simulink model "plant"  (R2014a)
settings: Solver=ode45  StartTime=0.0  StopTime=simTime  MaxStep=0.001  RelTol=1e-3
settings Model: Creator=Ash  LastModifiedBy=Ash
settings DataIOCC: ExternalInput=Input  LimitDataPoints=off  LoadExternalInput=on  OutputSaveName=r, r_d, s, s_d, r_dd, s_dd

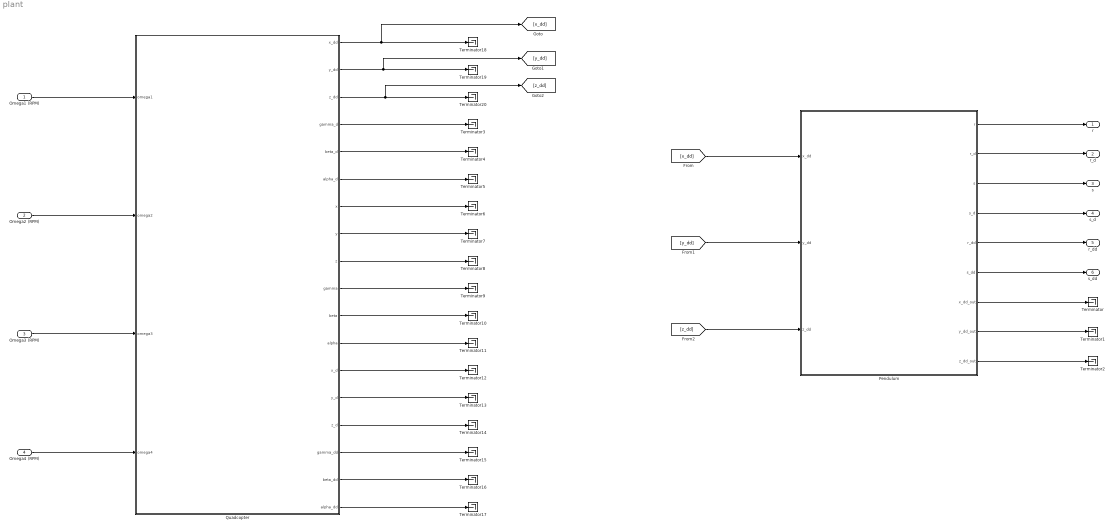
== system plant ==
  Omega1 (RPM) : Inport
  Omega2 (RPM) : Inport  Port=2
  Omega3 (RPM) : Inport  Port=3
  Omega4 (RPM) : Inport  Port=4
  Pendulum : Subsystem
  Quadcopter : Subsystem
  Terminator{,1..20} (21 alike) : Terminator
  r : Outport
  r_d : Outport  Port=2
  s : Outport  Port=3
  s_d : Outport  Port=4
  r_dd : Outport  Port=5
  s_dd : Outport  Port=6
  wires:
  Quadcopter/1(x_dd) -> Terminator18/1, [x_dd]
  Quadcopter/2(y_dd) -> Terminator19/1, [y_dd]
  Omega1 (RPM)/1 -> Quadcopter/1(omega1)
  Omega2 (RPM)/1 -> Quadcopter/2(omega2)
  Omega3 (RPM)/1 -> Quadcopter/3(omega3)
  Omega4 (RPM)/1 -> Quadcopter/4(omega4)
  Quadcopter/3(z_dd) -> Terminator20/1, [z_dd]
  Pendulum/1(r) -> r/1
  Pendulum/2(r_d) -> r_d/1
  Pendulum/4(s_d) -> s_d/1
  Pendulum/3(s) -> s/1
  Pendulum/5(r_dd) -> r_dd/1
  Pendulum/6(s_dd) -> s_dd/1
  [x_dd] -> Pendulum/1(x_dd)
  [y_dd] -> Pendulum/2(y_dd)
  [z_dd] -> Pendulum/3(z_dd)
  Pendulum/7(x_dd_out) -> Terminator/1
  Pendulum/9(z_dd_out) -> Terminator2/1
  Pendulum/8(y_dd_out) -> Terminator1/1
  Quadcopter/4(gamma_d) -> Terminator3/1
  Quadcopter/18(alpha_dd) -> Terminator17/1
  Quadcopter/17(beta_dd) -> Terminator16/1
  Quadcopter/16(gamma_dd) -> Terminator15/1
  Quadcopter/15(z_d) -> Terminator14/1
  Quadcopter/14(y_d) -> Terminator13/1
  Quadcopter/13(x_d) -> Terminator12/1
  Quadcopter/12(alpha) -> Terminator11/1
  Quadcopter/11(beta) -> Terminator10/1
  Quadcopter/10(gamma) -> Terminator9/1
  Quadcopter/9(z) -> Terminator8/1
  Quadcopter/8(y) -> Terminator7/1
  Quadcopter/7(x) -> Terminator6/1
  Quadcopter/6(alpha_d) -> Terminator5/1
  Quadcopter/5(beta_d) -> Terminator4/1

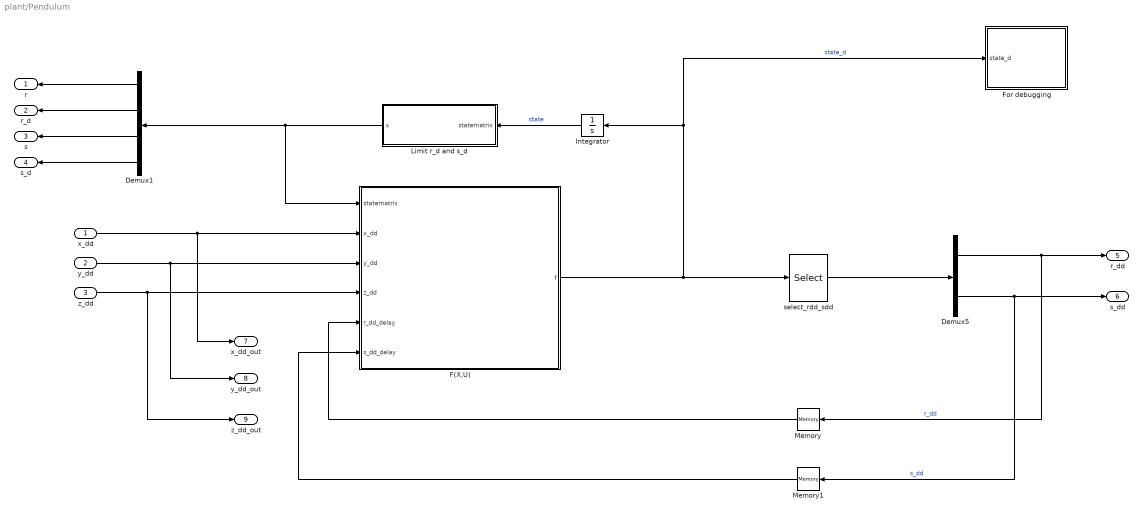
== system plant/Pendulum ==
  x_dd : Inport
  y_dd : Inport  Port=2
  z_dd : Inport  Port=3
  Demux1 : Demux  Outputs=[1 1 1 1]
  Demux5 : Demux  Outputs=[1 1]
  F(X,U) : MATLAB Function  TreatAsAtomicUnit=on
  For debugging : Subsystem
  Integrator : Integrator
  Limit r_d and s_d : MATLAB Function  TreatAsAtomicUnit=on
  Memory : Memory
  Memory1 : Memory
  select_rdd_sdd : Selector  InputPortWidth=4  Indices=[2 4]
  r : Outport
  r_d : Outport  Port=2
  s : Outport  Port=3
  s_d : Outport  Port=4
  r_dd : Outport  Port=5
  s_dd : Outport  Port=6
  x_dd_out : Outport  Port=7
  y_dd_out : Outport  Port=8
  z_dd_out : Outport  Port=9
  wires:
  Memory1/1 -> F(X,U)/6(s_dd_delay)
  Demux5/1 -> r_dd/1, Memory/1  "r_dd"
  Memory/1 -> F(X,U)/5(r_dd_delay)
  select_rdd_sdd/1 -> Demux5/1
  Demux5/2 -> s_dd/1, Memory1/1  "s_dd"
  z_dd/1 -> F(X,U)/4(z_dd), z_dd_out/1
  y_dd/1 -> F(X,U)/3(y_dd), y_dd_out/1
  Demux1/1 -> r/1
  Demux1/2 -> r_d/1
  Demux1/4 -> s_d/1
  Demux1/3 -> s/1
  F(X,U)/1(f) -> For debugging/1(state_d), Integrator/1, select_rdd_sdd/1  "state_d"
  x_dd/1 -> F(X,U)/2(x_dd), x_dd_out/1
  Limit r_d and s_d/1(x) -> F(X,U)/1(statematrix), Demux1/1
  Integrator/1 -> Limit r_d and s_d/1(statematrix)  "state"

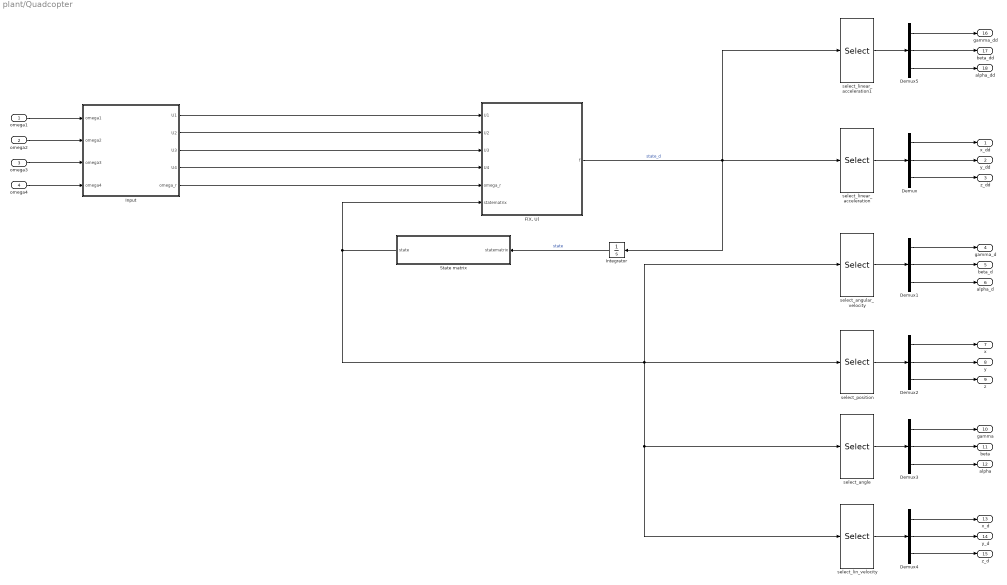
== system plant/Quadcopter ==
  omega1 : Inport
  omega2 : Inport  Port=2
  omega3 : Inport  Port=3
  omega4 : Inport  Port=4
  Demux{,1..5} (6 alike) : Demux  Outputs=[1 1 1]
  "F(X, U)" : MATLAB Function  TreatAsAtomicUnit=on
  Input : MATLAB Function  TreatAsAtomicUnit=on
  Integrator : Integrator
  State matrix : MATLAB Function  TreatAsAtomicUnit=on
  select_angle : Selector  InputPortWidth=12  Indices=[7 9 11]
  select_angular_velocity : Selector  InputPortWidth=12  Indices=[8 10 12]
  select_lin_velocity : Selector  InputPortWidth=12  Indices=[2 4 6]
  select_linear_acceleration : Selector  InputPortWidth=12  Indices=[2 4 6]
  select_linear_acceleration1 : Selector  InputPortWidth=12  Indices=[8 10 12]
  select_position : Selector  InputPortWidth=12  Indices=[1 3 5]
  x_dd : Outport
  y_dd : Outport  Port=2
  z_dd : Outport  Port=3
  gamma_d : Outport  Port=4
  beta_d : Outport  Port=5
  alpha_d : Outport  Port=6
  x : Outport  Port=7
  y : Outport  Port=8
  z : Outport  Port=9
  gamma : Outport  Port=10
  beta : Outport  Port=11
  alpha : Outport  Port=12
  x_d : Outport  Port=13
  y_d : Outport  Port=14
  z_d : Outport  Port=15
  gamma_dd : Outport  Port=16
  beta_dd : Outport  Port=17
  alpha_dd : Outport  Port=18
  wires:
  omega3/1 -> Input/3(omega3)
  omega2/1 -> Input/2(omega2)
  omega1/1 -> Input/1(omega1)
  select_linear_acceleration/1 -> Demux/1
  Demux/1 -> x_dd/1
  Demux/2 -> y_dd/1
  Demux/3 -> z_dd/1
  select_angular_velocity/1 -> Demux1/1
  Demux1/1 -> gamma_d/1
  Demux1/2 -> beta_d/1
  Demux1/3 -> alpha_d/1
  select_position/1 -> Demux2/1
  Demux2/1 -> x/1
  Demux2/2 -> y/1
  Demux2/3 -> z/1
  select_angle/1 -> Demux3/1
  Demux3/1 -> gamma/1
  Demux3/2 -> beta/1
  Demux3/3 -> alpha/1
  Integrator/1 -> State matrix/1(statematrix)  "state"
  select_lin_velocity/1 -> Demux4/1
  Demux4/1 -> x_d/1
  Demux4/2 -> y_d/1
  Demux4/3 -> z_d/1
  omega4/1 -> Input/4(omega4)
  Input/1(U1) -> "F(X, U)"/1(U1)
  Input/2(U2) -> "F(X, U)"/2(U2)
  Input/3(U3) -> "F(X, U)"/3(U3)
  Input/4(U4) -> "F(X, U)"/4(U4)
  Input/5(omega_r) -> "F(X, U)"/5(omega_r)
  "F(X, U)"/1(f) -> select_linear_acceleration1/1, select_linear_acceleration/1, Integrator/1  "state_d"
  select_linear_acceleration1/1 -> Demux5/1
  Demux5/1 -> gamma_dd/1
  Demux5/2 -> beta_dd/1
  Demux5/3 -> alpha_dd/1
  State matrix/1(state) -> "F(X, U)"/6(statematrix), select_angular_velocity/1, select_position/1, select_lin_velocity/1, select_angle/1

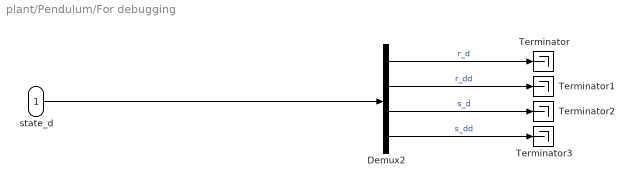
== system plant/Pendulum/For debugging ==
  state_d : Inport
  Demux2 : Demux  Outputs=[1 1 1 1]
  Terminator{,1..3} (4 alike) : Terminator
  wires:
  Demux2/4 -> Terminator3/1  "s_dd"
  Demux2/3 -> Terminator2/1  "s_d"
  Demux2/2 -> Terminator1/1  "r_dd"
  Demux2/1 -> Terminator/1  "r_d"
  state_d/1 -> Demux2/1

== matlab function plant/Quadcopter/State matrix ==
  data: state output; statematrix input
function state = fcn(statematrix)

x = statematrix(1);
x_d = statematrix(2);
y = statematrix(3);
y_d = statematrix(4);
z = statematrix(5);
z_d = statematrix(6);
gamma1 = statematrix(7);
gamma_d = statematrix(8);
beta1 = statematrix(9);
beta_d = statematrix(10);
alpha1 = statematrix(11);
alpha_d = statematrix(12);

gamma = mod(gamma1, 2*3.1416);
beta = mod(beta1, 2*3.1416);
alpha = mod(alpha1, 2*3.1416);

state = [x; x_d; y; y_d; z; z_d; gamma; gamma_d; beta; beta_d; alpha; alpha_d];

== matlab function plant/Quadcopter/F(X, U) ==
  data: U1 input; f output; U2 input; U3 input; U4 input; omega_r input; statematrix input
function f = fcn(U1, U2, U3, U4, omega_r, statematrix)

%syms b d
%syms l_qa l_r m_arm m_body m_rotor h_a h_b h_r r

g = -9.81;
l_qa = 0.25;
l_r = 0.1;
m_arm = 0.01;
m_body = 0.5;
m_rotor = 0.05;
h_a = 0.0025;
h_b = 0.05;
h_r = 0.001;
r = 0.025;

m = m_arm + m_body;
Ixx = (4*m_arm/3) * (h_a^3*(l_qa-r) + h_a*(l_qa^3 - r^3)) + (m_body/3) * (r^3*h_b + r*h_b^3);
Iyy = Ixx;
Izz = (8*m_arm/3) * (l_qa^4 + r^4 - l_qa^3*r - l_qa*r^3) + (2*m_body/3)*r^4;

%Ix = [Ixx 0 0; 0 0 0; 0 0 0];
%Iy = [0 0 0; 0 Iyy 0; 0 0 0];
%Iz = [0 0 0; 0 0 0; 0 0 Izz];
%J = Ix + Iy + Iz;  
Ix = Ixx;
Iy = Iyy;
Iz = Izz;             
J = [Ixx 0 0; 0 Iyy 0; 0 0 Izz];                        % inertia tensor of quadcopter
Jr_x = (m_rotor/3)*(l_r^3*h_r + l_r*h_r^3);
Jr_y = (m_rotor/3)*(l_r^3*h_r + l_r*h_r^3);
Jr_z = (2*m_rotor/3)*l_r^4;
Jr_vector = 4*[Jr_x 0 0; 0 Jr_y 0; 0 0 Jr_z];           % intertia tensor of all 4 rotors
Jr = sqrt(Jr_vector(1,1)^2 + Jr_vector(2,2)^2 + Jr_vector(3,3)^2);

x = statematrix(1);
x_d = statematrix(2);
y = statematrix(3);
y_d = statematrix(4);
z = statematrix(5);
z_d = statematrix(6);
gamma1 = statematrix(7);
gamma_d = statematrix(8);
beta1 = statematrix(9);
beta_d = statematrix(10);
alpha1 = statematrix(11);
alpha_d = statematrix(12);

gamma = mod(gamma1, 2*3.1416);
beta = mod(beta1, 2*3.1416);
alpha = mod(alpha1, 2*3.1416);

L_vector = mtimes(J, [gamma_d; beta_d; alpha_d]);
L = sqrt(L_vector(1)^2 + L_vector(2)^2 + L_vector(3)^2);

f = [x_d; -U1/m*(cos(gamma)*sin(beta)*cos(alpha) + sin(gamma)*sin(alpha)); y_d; -U1/m * (cos(gamma)*sin(alpha)*sin(beta) - sin(gamma)*cos(alpha)); z_d; ((U1/m)*cos(beta)*cos(gamma) + g); gamma_d; (beta_d*alpha_d*((Iy-Iz)/Ix) - (Jr/Ix)*beta_d*omega_r + (L/Ix)*U2); beta_d; (gamma_d*alpha_d*((Iz-Ix)/Iy) + (Jr/Iy)*gamma_d*omega_r + (L/Iy)*U3); alpha_d; (gamma_d*beta_d*((Ix-Iy)/Iz) + (1/Iz)*U4)];

== matlab function plant/Quadcopter/Input ==
  data: omega1 input; omega2 input; omega3 input; U1 output; omega4 input; U2 output; U3 output; U4 output; omega_r output
function [U1, U2, U3, U4, omega_r] = fcn(omega1, omega2 ,omega3, omega4)

%syms b d
b = 3.13e-5;
d = 9e-7;

% convert to rad/s
o1 = omega1 * 2 * pi / 60;
o2 = omega2 * 2 * pi / 60;
o3 = omega3 * 2 * pi / 60;
o4 = omega4 * 2 * pi / 60;

U1 = b*(o1^2 + o2^2 + o3^2 + o4^2);
U2 = b*(-o2^2 + o4^2);
U3 = b*(o1^2 - o3^2);
U4 = d*(o1^2 - o2^2 + o3^2 - o4^2);
omega_r = -o1 + o2 - o3 + o4;

== matlab function plant/Pendulum/F(X,U) ==
  data: statematrix input; x_dd input; y_dd input; z_dd input; r_dd_delay input; s_dd_delay input; f output
function f = fcn(statematrix, x_dd, y_dd, z_dd, r_dd_delay, s_dd_delay)

g = -9.81;
L = 0.4;

r = statematrix(1);
r_d = statematrix(2);
s = statematrix(3);
s_d = statematrix(4);

if ((r^2 + s^2) <= (L^2))
    
    zeta = sqrt(L^2 - r^2 - s^2);
    r_dd = (1/((L^2 - s^2)*zeta)) * ( -r^4*x_dd - (L^2 - s^2)^2*x_dd - 2*r^2*(s*r_d*s_d + (-L^2 + s^2)*x_dd) + r^3*(s_d^2 + s*s_dd_delay - zeta*(g+z_dd)) + r*(-L^2*s*s_dd_delay + s^3*s_dd_delay + s^2*(r_d^2 - zeta*(g+z_dd)) + L^2*(-r_d^2 - s_d^2 + zeta*(g+z_dd))) );
    s_dd = (1/((L^2 - r^2)*zeta)) * ( -s^4*y_dd - (L^2 - r^2)^2*y_dd - 2*s^2*(r*r_d*s_d + (-L^2 + r^2)*y_dd) + s^3*(r_d^2 + r*r_dd_delay - zeta*(g+z_dd)) + s*(-L^2*r*r_dd_delay + r^3*r_dd_delay + r^2*(s_d^2 - zeta*(g+z_dd)) + L^2*(-r_d^2 - s_d^2 + zeta*(g+z_dd))) );

    
else
    
    r_d = 0;
    s_d = 0;
    r_dd = 0;
    s_dd = 0;
    
end


f = [r_d; r_dd; s_d; s_dd];

== matlab function plant/Pendulum/Limit r_d and s_d ==
  data: statematrix input; x output
function x = fcn(statematrix)

L = 0.4;

r = statematrix(1);
r_d = statematrix(2);
s = statematrix (3);
s_d = statematrix(4);

if ((r^2 + s^2) > (L^2))
    
    r_d = 0;
    s_d = 0;
    
end

x = [r; r_d; s; s_d];
